simulink library "rwa_assembly_lib"  (R2018b)
settings: Solver=VariableStepAuto  StartTime=0.0  StopTime=10.0  RelTol=1e-3
undefined symbols (not defined in the file): simParams
libraries: rw_motor_lib x4
settings Model: Creator=Taylor  LastModifiedBy=colem

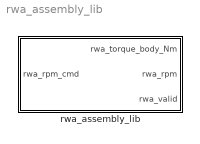
== system rwa_assembly_lib ==
  rwa_assembly_lib : Subsystem

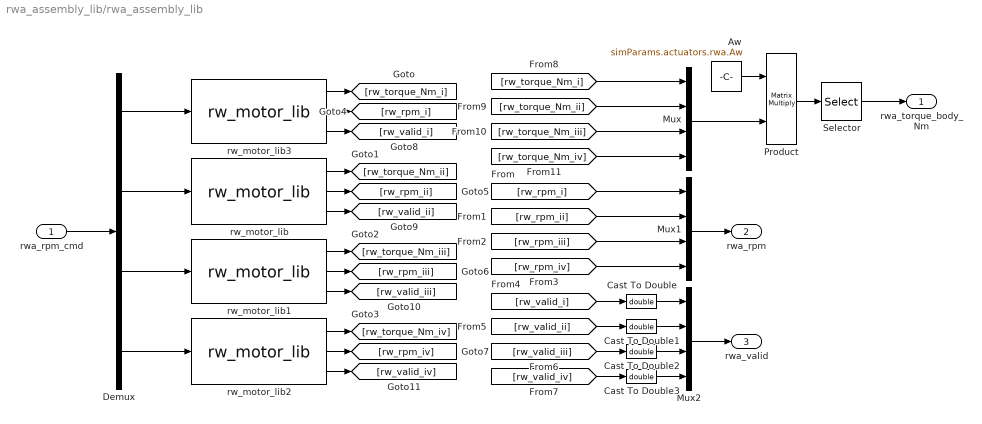
== system rwa_assembly_lib/rwa_assembly_lib ==
  rwa_rpm_cmd : Inport
  Aw : Constant  Value=simParams.actuators.rwa.Aw
  Cast To Double{,1..3} (4 alike) : DataTypeConversion  OutDataTypeStr=double
  Demux : Demux
  Mux : Mux
  Mux1 : Mux
  Mux2 : Mux
  Product : Product  Multiplication=Matrix(*)
  Selector : Selector  InputPortWidth=4  IndexOptions=Index vector (dialog)  Indices=[1 2 3]  OutputSizes=1
  rw_motor_lib : rw_motor_lib/rw_motor_lib  id_a=2
  rw_motor_lib1 : rw_motor_lib/rw_motor_lib  id_a=3
  rw_motor_lib2 : rw_motor_lib/rw_motor_lib  id_a=4
  rw_motor_lib3 : rw_motor_lib/rw_motor_lib  id_a=1
  rwa_torque_body_Nm : Outport
  rwa_rpm : Outport  Port=2
  rwa_valid : Outport  Port=3
  wires:
  rwa_rpm_cmd/1 -> Demux/1
  Demux/1 -> rw_motor_lib3/1
  Demux/2 -> rw_motor_lib/1
  Demux/3 -> rw_motor_lib1/1
  Demux/4 -> rw_motor_lib2/1
  rw_motor_lib3/1 -> [rw_torque_Nm_i]
  rw_motor_lib/1 -> [rw_torque_Nm_ii]
  rw_motor_lib1/1 -> [rw_torque_Nm_iii]
  rw_motor_lib2/1 -> [rw_torque_Nm_iv]
  rw_motor_lib3/2 -> [rw_rpm_i]
  rw_motor_lib/2 -> [rw_rpm_ii]
  rw_motor_lib1/2 -> [rw_rpm_iii]
  rw_motor_lib2/2 -> [rw_rpm_iv]
  Mux/1 -> Product/2
  Mux1/1 -> rwa_rpm/1
  [rw_rpm_i] -> Mux1/1
  [rw_rpm_ii] -> Mux1/2
  rw_motor_lib3/3 -> [rw_valid_i]
  rw_motor_lib/3 -> [rw_valid_ii]
  rw_motor_lib1/3 -> [rw_valid_iii]
  rw_motor_lib2/3 -> [rw_valid_iv]
  [rw_rpm_iii] -> Mux1/3
  [rw_rpm_iv] -> Mux1/4
  Mux2/1 -> rwa_valid/1
  [rw_valid_iv] -> Cast To Double3/1
  [rw_valid_ii] -> Cast To Double1/1
  [rw_valid_iii] -> Cast To Double2/1
  [rw_valid_i] -> Cast To Double/1
  Aw/1 -> Product/1
  Product/1 -> Selector/1
  Selector/1 -> rwa_torque_body_Nm/1
  [rw_torque_Nm_i] -> Mux/1
  [rw_torque_Nm_ii] -> Mux/2
  [rw_torque_Nm_iii] -> Mux/3
  [rw_torque_Nm_iv] -> Mux/4
  Cast To Double/1 -> Mux2/1
  Cast To Double1/1 -> Mux2/2
  Cast To Double2/1 -> Mux2/3
  Cast To Double3/1 -> Mux2/4
